simulink model "RLC_simulink"  (R2024b)
settings: Solver=VariableStepAuto  StartTime=0.0  StopTime=0.002  RelTol=1e-3
InitFcn:
  | R=120;
  | L=0.006;
  | C=0.0000001;

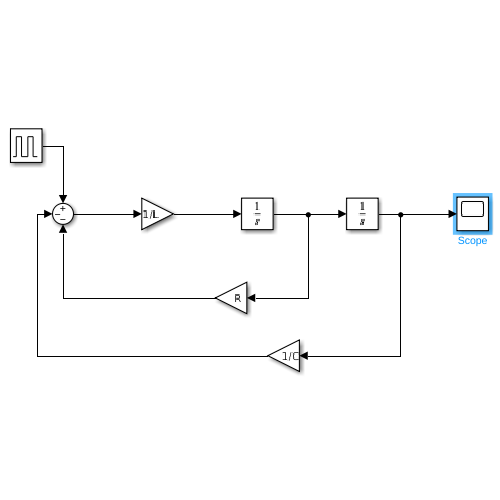
[thumbnail: Simulink's stored preview of the top-level diagram]
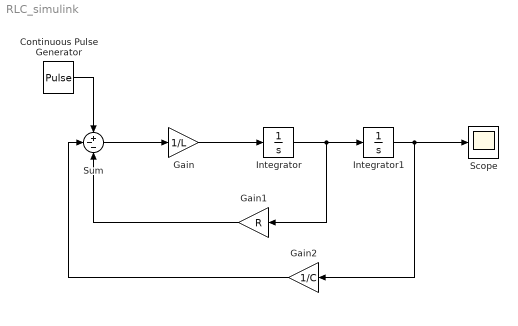
== system RLC_simulink ==
  Continuous Pulse Generator : DiscretePulseGenerator  PulseType=Time based  Amplitude=5  Period=0.002  PulseWidth=50
  Gain : Gain  Gain=1/L
  Gain1 : Gain  Gain=R
  Gain2 : Gain  Gain=1/C
  Integrator : Integrator
  Integrator1 : Integrator
  Scope : Scope
  Sum : Sum  Inputs=+--
  wires:
  Integrator/1 -> Gain1/1, Integrator1/1
  Gain/1 -> Integrator/1
  Integrator1/1 -> Gain2/1, Scope/1
  Gain1/1 -> Sum/3
  Gain2/1 -> Sum/2
  Continuous Pulse Generator/1 -> Sum/1
  Sum/1 -> Gain/1
